simulink library "hal"  (Simulink 8.2)
settings: Solver=ode45  SolverMode=SingleTasking  StartTime=0.0  StopTime=10.0  RelTol=1e-3
PostLoadFcn:
  | , if any(exist('dsrtsu_mdlpostloadfcn', 'file') == [2, 3, 6]), try dsrtsu_mdlpostloadfcn('Execute', bdroot); catch fprintf('Error in PostLoadFcn (dsrtsu_mdlpostloadfcn) for model "%s":\n %s\n', bdroot, lasterr); end, end,
values from neighbouring files (symbols this model uses):
  INVALID_ABS1_TIMEOUT = single(0.03)    [hal_def.m]
  INVALID_ABS2_TIMEOUT = single(0.03)    [hal_def.m]
  INVALID_ABS3_TIMEOUT = single(0.03)    [hal_def.m]
  INVALID_ABS4_TIMEOUT = single(0.03)    [hal_def.m]
  INVALID_AC1_TIMEOUT = single(0.3)    [hal_def.m]
  INVALID_BCM1_TIMEOUT = single(0.6)    [hal_def.m]
  INVALID_BCM2_TIMEOUT = single(0.06)    [hal_def.m]
  INVALID_BOOSTER_VAC = uint32(255)    [hal_def.m]
  INVALID_CUR_VEHDECE = uint32(255)    [hal_def.m]
  INVALID_CURBRAKEDECE_REQ = uint32(255)    [hal_def.m]
  INVALID_CURSTEERANG_REQ = uint32(65535)    [hal_def.m]
  INVALID_CURSTEERTQ_REQ = uint32(255)    [hal_def.m]
  INVALID_ECM1_TIMEOUT = single(0.03)    [hal_def.m]
  INVALID_ECM2_TIMEOUT = single(0.03)    [hal_def.m]
  INVALID_ECM3_TIMEOUT = single(0.03)    [hal_def.m]
  INVALID_ECM9_TIMEOUT = single(0.03)    [hal_def.m]
  INVALID_ENG_TORQUE_FRICTIONAL = uint32(255)    [hal_def.m]
  INVALID_ENG_TORQUE_INDICATED = uint32(255)    [hal_def.m]
  INVALID_ENG_TORQUE_INDICATEDCOR = uint32(255)    [hal_def.m]
  INVALID_ENG_TQ_MAX = uint32(65535)    [hal_def.m]
  INVALID_ENG_TQ_MIN = uint32(65535)    [hal_def.m]
  INVALID_EPAS2_TIMEOUT = single(0.03)    [hal_def.m]
  INVALID_EPAS3_TIMEOUT = single(0.03)    [hal_def.m]
  INVALID_EPB1_TIMEOUT = single(0.12)    [hal_def.m]
  INVALID_EPS_BATTVOLT = uint32(251)    [hal_def.m]
  INVALID_ESC_BATTVOLT = uint32(251)    [hal_def.m]
  INVALID_GRADE = uint32(255)    [hal_def.m]
  INVALID_HCU3_TIMEOUT = single(0.03)    [hal_def.m]
  INVALID_HCU4_TIMEOUT = single(0.03)    [hal_def.m]
  INVALID_HMI1_TIMEOUT = single(0.03)    [hal_def.m]
  INVALID_HMI2_TIMEOUT = single(0.03)    [hal_def.m]
  INVALID_LAT_ACC = uint32(255)    [hal_def.m]
  INVALID_LONG_ACC = uint32(255)    [hal_def.m]
  INVALID_MC_PRESSURE = uint32(2047)    [hal_def.m]
  INVALID_METER1_TIMEOUT = single(0.3)    [hal_def.m]
  INVALID_METER3_TIMEOUT = single(0.3)    [hal_def.m]
  INVALID_METER_VEHSPD = uint32(2048)    [hal_def.m]
  INVALID_ODO_METER = uint32(1000000)    [hal_def.m]
  INVALID_OUTSIDE_TEMP = uint32(96)    [hal_def.m]
  INVALID_PARKBRAKEBIND_STAT = uint32(3)    [hal_def.m]
  INVALID_SAS1_TIMEOUT = single(0.03)    [hal_def.m]
  INVALID_SAS_ANGLE = uint32(65535)    [hal_def.m]
  INVALID_SHIFTER_POSN = uint32(6)    [hal_def.m]
  INVALID_TCM1_TIMEOUT = single(0.03)    [hal_def.m]
  INVALID_TCM2_TIMEOUT = single(0.03)    [hal_def.m]
  INVALID_VCU1_TIMEOUT = single(0.03)    [hal_def.m]
  INVALID_VCU2_TIMEOUT = single(0.03)    [hal_def.m]
  INVALID_VEH_CRASH = uint32(15)    [hal_def.m]
  INVALID_VEH_SPD = uint32(2048)    [hal_def.m]
  INVALID_WHEEL_SPD = uint32(16377)    [hal_def.m]
  INVALID_YAW_RATE = uint32(2001)    [hal_def.m]
undefined symbols (not defined in the file or in its folder): C_TASK_5MS_S, FALSE, INVALID_CURPTTORQ_REQ, KHAL_MssgIdObj1_num, KHAL_MssgIdObj2_num, KHAL_MssgIdObjStatus_num, TRUE
libraries: simulink x92
(part 1 of 8)
settings Model: DSRTSU_INTERNAL_RTI_VER=460  DSRTSU_INTERNAL_RTI_TYPE=rti1401  RTICANMMDATA=struct('GeneralSetupData',struct('modelroot','D:\HAITEC\SVN\trunk\ADAS_Softwares\HTDragon\software\sw_development\arch\hal','generalsettings',struct('filesettings',struct('destfolder',struct('Name','RTICANMM_FILES','Check',1),'buildfolder',struct('Name','.','Check',1),'AbsDestfolder',struct('Name','D:\HAITEC\SVN\trunk\ADAS_Softwares\HTDragon\software\sw_development\arch\hal\RTICANMM_FILES'),'AbsBuildfolder',struct('Name','D:\HAITEC\SVN\trunk\ADAS_Softwares\HTDragon\software\sw_development\arch\hal'))),'options',struct('addpaths',1,'rmpaths',1,'addtrcexclusion',logical(1),'cannavigator',struct('checkmonitoring',0),'show_usrtrc',0,'use_usrtrc',0),'advanced',struct('options',[1 1 1 1 1 1 1 1 1 1 1 1 1 1 1 1 1 1 1 1 1 1 1 1 1 1 1 1 1 1 1 1 1 1 1 1 1 1 1 1 1 1 1 1 1 1 1 1 1 1 1 1 1 1 1 1 1 1 1 1 1 1 1 1 1 1 1 1 1 1 1 1 1 1 1 1 1 1 1 1 1 1 1 1 1 1 1 1 1 1 1 1 1 1 1 1 1 1 1 1]),'MPSetup',{{}},'modelname','hal','block','hal'))  DSRTSU_INTERNAL_RTIFPGA=50  Creator=WX  LastModifiedBy=14014

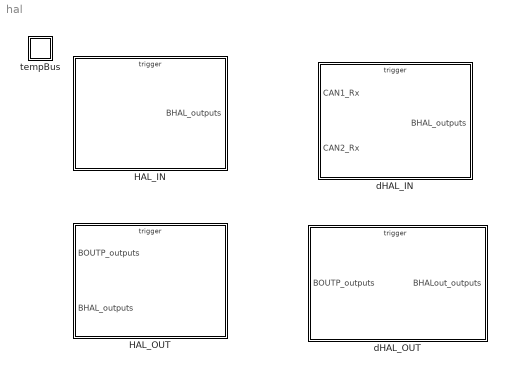
== system hal ==
  HAL_IN : Subsystem
  HAL_OUT : Subsystem  TreatAsAtomicUnit=on
      settings: RTWSystemCode=Nonreusable function  RTWFcnNameOpts=Use subsystem name  RTWFileNameOpts=Use subsystem name
  dHAL_IN : Subsystem
  dHAL_OUT : Subsystem  TreatAsAtomicUnit=on
      settings: RTWSystemCode=Nonreusable function  RTWFcnNameOpts=Use subsystem name  RTWFileNameOpts=Use subsystem name
  tempBus : Subsystem

== system hal/HAL_IN ==
  trig_hal_in : TriggerPort  TriggerType=function-call
  ADCFaultCvt : DataTypeConversion  OutDataTypeStr=uint8  SaturateOnIntegerOverflow=on  RndMeth=Zero
  AppTimeCvt : DataTypeConversion  OutDataTypeStr=single  SaturateOnIntegerOverflow=on  RndMeth=Zero
  EEPROMFaultCvt : DataTypeConversion  OutDataTypeStr=uint8  SaturateOnIntegerOverflow=on  RndMeth=Zero
  Ground{,1..8} (9 alike) : Ground
  IgnitionVoltCvt : DataTypeConversion  OutDataTypeStr=single  SaturateOnIntegerOverflow=on  RndMeth=Zero
  IgnitionVoltCvt1 : DataTypeConversion  OutDataTypeStr=single  SaturateOnIntegerOverflow=on  RndMeth=Zero
  RAMFaultCvt : DataTypeConversion  OutDataTypeStr=uint8  SaturateOnIntegerOverflow=on  RndMeth=Zero
  ROMFaultCvt : DataTypeConversion  OutDataTypeStr=uint8  SaturateOnIntegerOverflow=on  RndMeth=Zero
  VREF1FaultCvt : DataTypeConversion  OutDataTypeStr=uint8  SaturateOnIntegerOverflow=on  RndMeth=Zero
  VREF2FaultCvt : DataTypeConversion  OutDataTypeStr=uint8  SaturateOnIntegerOverflow=on  RndMeth=Zero
  halbus : BusCreator  Inputs=9  OutDataTypeStr=Bus: BHAL_outputs
  BHAL_outputs : Outport  OutDataTypeStr=Bus: BHAL_outputs
  wires:
  IgnitionVoltCvt/1 -> halbus/1  "VHAL_IgnitionVolt_V"
  AppTimeCvt/1 -> halbus/3  "VHAL_AppTime_ms"
  ADCFaultCvt/1 -> halbus/4  "VHAL_ADCFault_enum"
  EEPROMFaultCvt/1 -> halbus/5  "VHAL_EEPROMFault_enum"
  RAMFaultCvt/1 -> halbus/6  "VHAL_RAMFault_enum"
  ROMFaultCvt/1 -> halbus/7  "VHAL_ROMFault_enum"
  VREF1FaultCvt/1 -> halbus/8  "VHAL_VREF1Fault_enum"
  VREF2FaultCvt/1 -> halbus/9  "VHAL_VREF2Fault_enum"
  IgnitionVoltCvt1/1 -> halbus/2  "VHAL_VbatprotVolt_V"
  halbus/1 -> BHAL_outputs/1  "BHAL_outputs"
  Ground/1 -> IgnitionVoltCvt/1
  Ground1/1 -> IgnitionVoltCvt1/1
  Ground2/1 -> AppTimeCvt/1
  Ground3/1 -> ADCFaultCvt/1
  Ground4/1 -> EEPROMFaultCvt/1
  Ground5/1 -> RAMFaultCvt/1
  Ground6/1 -> ROMFaultCvt/1
  Ground7/1 -> VREF1FaultCvt/1
  Ground8/1 -> VREF2FaultCvt/1

== system hal/HAL_OUT ==
  BOUTP_outputs : Inport  OutDataTypeStr=Bus: BOUTP_outputs
  BHAL_outputs : Inport  Port=2  OutDataTypeStr=Bus: BHAL_outputs
  trig_hal_out : TriggerPort  TriggerType=function-call
  wires:
  BOUTP_outputs/1 -> [BOUTP_outputs]
  BHAL_outputs/1 -> [BHAL_outputs]
